simulink model "Oven_System"  (R2016a)
settings: Solver=VariableStepAuto  StartTime=0.0  StopTime=10.0  RelTol=1e-3
values from neighbouring files (symbols this model uses):
  Area = windowArea + wallArea    (= 5.25)    [Controller.m]
  c = 1005.4    [Controller.m]    (also in HighTrapMF.m = Points(3); LowTrapMF.m = Points(3); MAE_565_FuzzyLogic.m; TrapMF.m = Points(3))
  M = (lenOven*widOven*htOven)*densAir    (= 1.225)    [Controller.m]    (also in MAE_565_FuzzyLogic.m)
undefined symbols (not defined in the file or in its folder): Convert, Power, Req, sigbuilder_block
settings Model: Creator=levi.hubbard  LastModifiedBy=levi.hubbard

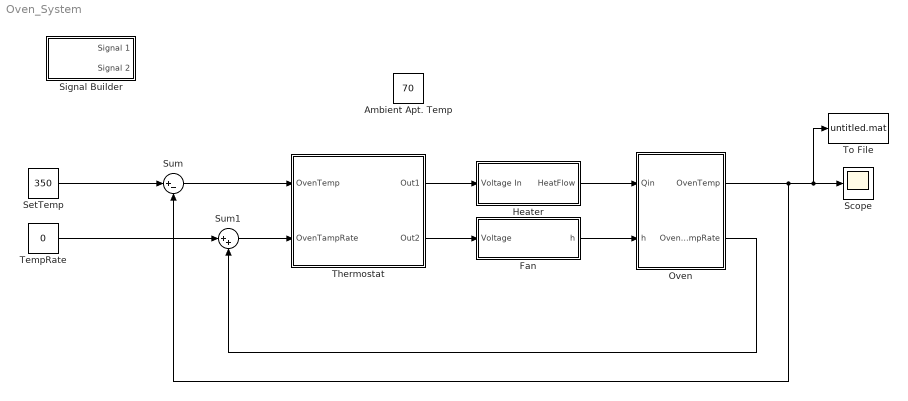
== system Oven_System ==
  "Ambient Apt. Temp " : Constant  Value=70
  Fan : Subsystem
  "Heater " : Subsystem
  "Oven " : Subsystem
  Scope : Scope
  SetTemp : Constant  Value=350
  Signal Builder : Subsystem  Tag=STV Subsys  LoadFcn=sigbuilder_block('load');  StartFcn=sigbuilder_block('start');  StopFcn=sigbuilder_block('stop');  ClipboardFcn=sigbuilder_block('clipboard');  mask(Sigbuilder block){}
      mask help: Simulink:masks:SigbuilderBlock_MD
      mask init:
      | if ~strcmp(get_param(bdroot(gcbh),'SimulationStatus'),'stopped') tuvar = sigbuilder_block('maskInit'); end
      settings: CopyFcn=sigbuilder_block('copy');  DeleteFcn=sigbuilder_block('delete');  ModelCloseFcn=sigbuilder_block('modelClose');  PreSaveFcn=sigbuilder_block('preSave');  PauseFcn=sigbuilder_block('pause');  ContinueFcn=sigbuilder_block('continue');  NameChangeFcn=sigbuilder_block('namechange');  OpenFcn=sigbuilder_block('open',[232.5 201 550.5 399.75 ]);  CloseFcn=sigbuilder_block('close');
      mask Display: plot(0, 0, 100, 100,[2, 2, 32, 32, 2], [68, 8, 8, 68, 68],[32, 2], [38, 38], [32, 19, 2],[53, 60, 44], [32, 17, 17, 2],[16, 16, 31, 31]);txt = getActiveGroup(gcbh);text(2, 100, txt,'verticalAlignment', 'top');
  Sum : Sum  Inputs=|+-
  Sum1 : Sum  Inputs=|++
  TempRate : Constant  Value=0
  Thermostat : Subsystem
  To File : ToFile  SaveFormat=Timeseries
  wires:
  SetTemp/1 -> Sum/1
  Sum/1 -> Thermostat/1(OvenTemp)
  Fan/1(h) -> "Oven "/2(h)
  "Heater "/1(HeatFlow) -> "Oven "/1(Qin)
  "Oven "/1(OvenTemp) -> To File/1, Scope/1, Sum/2
  Thermostat/1(Out1) -> "Heater "/1("Voltage In ")
  Thermostat/2(Out2) -> Fan/1(" Voltage ")
  TempRate/1 -> Sum1/1
  Sum1/1 -> Thermostat/2(OvenTampRate)
  "Oven "/2(OvenTempRate) -> Sum1/2

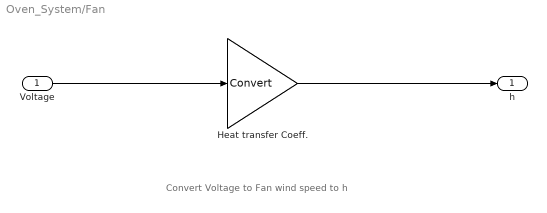
== system Oven_System/Fan ==
  note: Convert Voltage to Fan wind speed to h
  " Voltage " : Inport
  Heat transfer Coeff. : Gain  Gain=Convert
  h : Outport
  wires:
  " Voltage "/1 -> Heat transfer Coeff./1
  Heat transfer Coeff./1 -> h/1

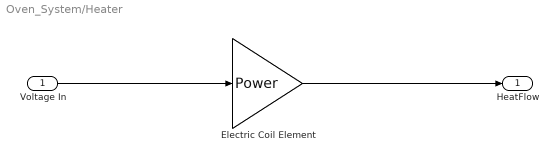
== system Oven_System/Heater  ==
  "Voltage In " : Inport
  Electric Coil Element : Gain  Gain=Power
  HeatFlow : Outport
  wires:
  "Voltage In "/1 -> Electric Coil Element/1
  Electric Coil Element/1 -> HeatFlow/1

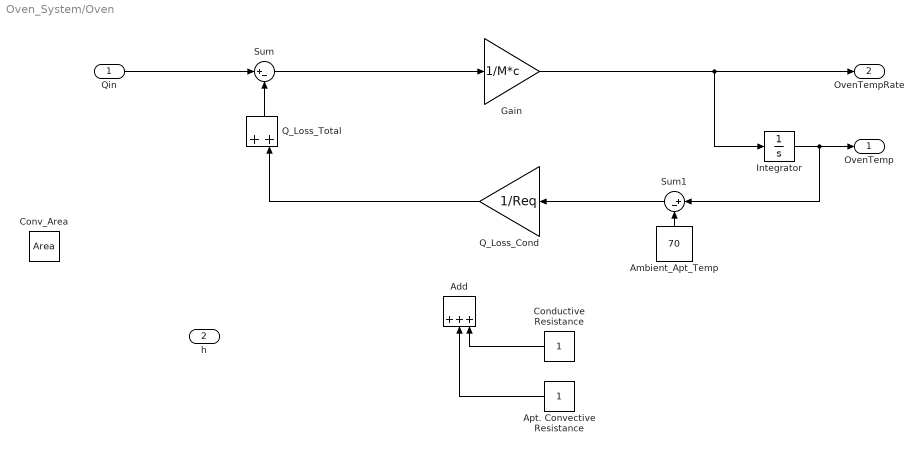
== system Oven_System/Oven  ==
  Qin : Inport
  h : Inport  Port=2
  " Apt. Convective Resistance" : Constant
  Add : Sum  Inputs=+++
  Ambient_Apt_Temp : Constant  Value=70
  Conductive Resistance : Constant
  Conv_Area : Constant  Value=Area
  Gain : Gain  Gain=1/M*c
  Integrator : Integrator
  Q_Loss_Cond : Gain  Gain=1/Req
  Q_Loss_Total : Sum
  Sum : Sum  Inputs=|+-
  Sum1 : Sum  Inputs=|+-
  OvenTemp : Outport
  OvenTempRate : Outport  Port=2
  wires:
  Sum/1 -> Gain/1
  Gain/1 -> OvenTempRate/1, Integrator/1
  Ambient_Apt_Temp/1 -> Sum1/2
  Q_Loss_Total/1 -> Sum/2
  Q_Loss_Cond/1 -> Q_Loss_Total/2
  Sum1/1 -> Q_Loss_Cond/1
  Qin/1 -> Sum/1
  Integrator/1 -> OvenTemp/1, Sum1/1
  Conductive Resistance/1 -> Add/3
  " Apt. Convective Resistance"/1 -> Add/2

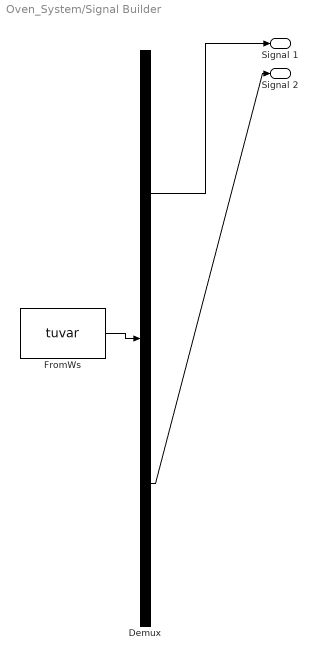
== system Oven_System/Signal Builder ==
  Demux : Demux  Tag=STV Demux  Outputs=2
  FromWs : FromWorkspace  Tag=STV FromWs  VariableName=tuvar  SampleTime=0
      SigBuilderData=|
      | common.afterFinalStr = 'Extrapolate'
      | common.sampleTime = '0'
      | dataSet.timeRange = [0 10]
      | dataSet.name = 'Group 1'
      | sbobj.Groups.Name = 'Group 1'
      | sbobj.Groups.Signals(1).Name = 'Signal 1'
      | sbobj.Groups.Signals(1).XData = [0 4 4 6 6 10]
      | sbobj.Groups.Signals(1).YData = [0 0 0.35 0.35 0.4 0.4]
      | sbobj.Groups.Signals(2).Name = 'Signal 2'
      | sbobj.Groups.Signals(2).XData = [0 5 5 10]
      | sbobj.Groups.Signals(2).YData = [0.4 0.4 0.35 0.35]
  Signal 1 : Outport  Tag=STV Outport
  Signal 2 : Outport  Tag=STV Outport  Port=2
  wires:
  Demux/1 -> Signal 1/1
  FromWs/1 -> Demux/1
  Demux/2 -> Signal 2/1

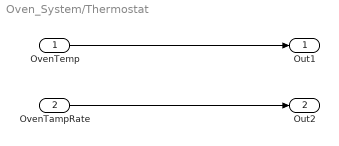
== system Oven_System/Thermostat ==
  OvenTemp : Inport
  OvenTampRate : Inport  Port=2
  Out1 : Outport
  Out2 : Outport  Port=2
  wires:
  OvenTemp/1 -> Out1/1
  OvenTampRate/1 -> Out2/1
